simulink model "klmn"  (R2023a)
settings: Solver=VariableStepAuto  StartTime=0.0  StopTime=10.0  RelTol=1e-3
values from neighbouring files (symbols this model uses):
  A = [0 1 0; 0 0 -1; 0 0 b_a]    [kalman_test.m]
  B = [0 1 0]'    [kalman_test.m]
  C = [1 0 0]    [kalman_test.m]
settings Model: Creator=xenja  LastModifiedBy=xenja

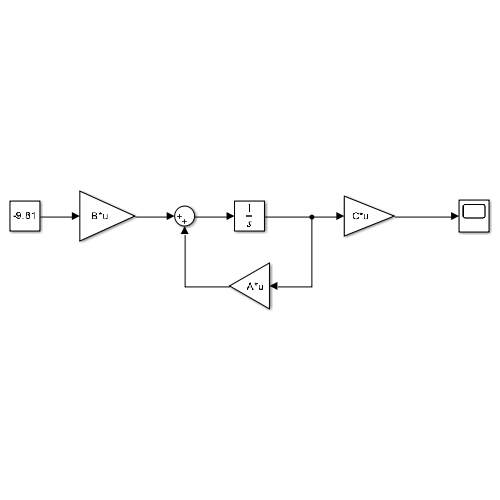
[thumbnail: Simulink's stored preview of the top-level diagram]
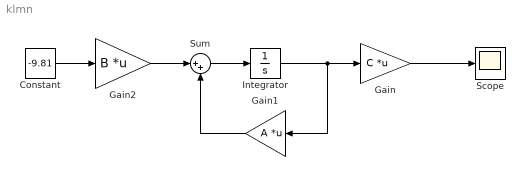
== system klmn ==
  Constant : Constant  Value=-9.81
  Gain : Gain  Gain=C  Multiplication=Matrix(K*u)
  Gain1 : Gain  Gain=A  Multiplication=Matrix(K*u)
  Gain2 : Gain  Gain=B  Multiplication=Matrix(K*u)
  Integrator : Integrator
  Scope : Scope
  Sum : Sum  Inputs=|++
  wires:
  Sum/1 -> Integrator/1
  Integrator/1 -> Gain/1, Gain1/1
  Gain1/1 -> Sum/2
  Gain2/1 -> Sum/1
  Constant/1 -> Gain2/1
  Gain/1 -> Scope/1
